simulink model "modelo_SEIR"  (R2019b)
settings: Solver=VariableStepAuto  StartTime=0.0  StopTime=360  RelTol=1e-3
settings Model: Creator=lucia  LastModifiedBy=lucia

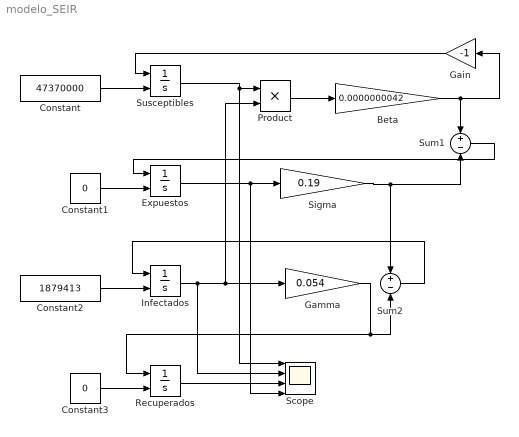
== system modelo_SEIR ==
  Beta : Gain  Gain=0.0000000042
  Constant : Constant  Value=47370000
  Constant1 : Constant  Value=0
  Constant2 : Constant  Value=1879413
  Constant3 : Constant  Value=0
  Expuestos : Integrator  InitialConditionSource=external
  Gain : Gain  Gain=-1
  Gamma : Gain  Gain=0.054
  Infectados : Integrator  InitialConditionSource=external
  Product : Product
  Recuperados : Integrator  InitialConditionSource=external
  Scope : Scope  NumInputPorts=4
  Sigma : Gain  Gain=0.19
  Sum1 : Sum  Inputs=+-
  Sum2 : Sum  Inputs=+-
  Susceptibles : Integrator  InitialConditionSource=external
  wires:
  Constant/1 -> Susceptibles/2
  Constant3/1 -> Recuperados/2
  Constant2/1 -> Infectados/2
  Constant1/1 -> Expuestos/2
  Susceptibles/1 -> Scope/1, Product/1
  Infectados/1 -> Scope/2, Product/2, Gamma/1
  Product/1 -> Beta/1
  Beta/1 -> Gain/1, Sum1/1
  Expuestos/1 -> Scope/4, Sigma/1
  Sigma/1 -> Sum2/1, Sum1/2
  Sum1/1 -> Expuestos/1
  Sum2/1 -> Infectados/1
  Recuperados/1 -> Scope/3
  Gamma/1 -> Recuperados/1, Sum2/2
  Gain/1 -> Susceptibles/1
